simulink model "ex4_enabled_triggered"  (R2021a)
settings: Solver=VariableStepAuto  StartTime=0.0  StopTime=10.0  RelTol=1e-3
settings Model: Creator=reemb  LastModifiedBy=reemb

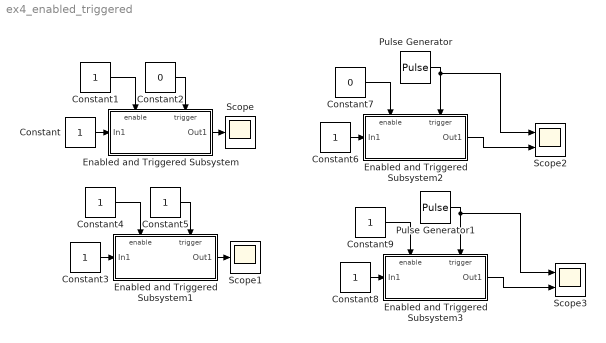
== system ex4_enabled_triggered ==
  Constant{,1,3..6,8..9} (8 alike) : Constant
  Constant2 : Constant  Value=0
  Constant7 : Constant  Value=0
  Enabled and Triggered Subsystem : Subsystem  TreatAsAtomicUnit=on
  Enabled and Triggered Subsystem1 : Subsystem  TreatAsAtomicUnit=on
  Enabled and Triggered Subsystem2 : Subsystem  TreatAsAtomicUnit=on
  Enabled and Triggered Subsystem3 : Subsystem  TreatAsAtomicUnit=on
  Pulse Generator : DiscretePulseGenerator  PulseType=Time based  PulseWidth=50
  Pulse Generator1 : DiscretePulseGenerator  PulseType=Time based  PulseWidth=50
  Scope : Scope
  Scope1 : Scope
  Scope2 : Scope  NumInputPorts=2
  Scope3 : Scope  NumInputPorts=2
  wires:
  Constant/1 -> Enabled and Triggered Subsystem/1(In1)
  Constant1/1 -> Enabled and Triggered Subsystem/Enable
  Constant2/1 -> Enabled and Triggered Subsystem/Trigger
  Enabled and Triggered Subsystem/1(Out1) -> Scope/1
  Enabled and Triggered Subsystem1/1(Out1) -> Scope1/1
  Constant5/1 -> Enabled and Triggered Subsystem1/Trigger
  Constant4/1 -> Enabled and Triggered Subsystem1/Enable
  Constant3/1 -> Enabled and Triggered Subsystem1/1(In1)
  Constant6/1 -> Enabled and Triggered Subsystem2/1(In1)
  Constant7/1 -> Enabled and Triggered Subsystem2/Enable
  Pulse Generator/1 -> Scope2/1, Enabled and Triggered Subsystem2/Trigger
  Enabled and Triggered Subsystem2/1(Out1) -> Scope2/2
  Enabled and Triggered Subsystem3/1(Out1) -> Scope3/2
  Pulse Generator1/1 -> Enabled and Triggered Subsystem3/Trigger, Scope3/1
  Constant9/1 -> Enabled and Triggered Subsystem3/Enable
  Constant8/1 -> Enabled and Triggered Subsystem3/1(In1)

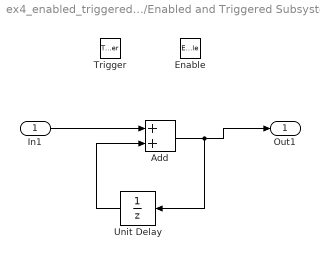
== system ex4_enabled_triggered/Enabled and Triggered Subsystem ==
  In1 : Inport
  Enable : EnablePort
  Trigger : TriggerPort  VariantControl=(inherit)
  Add : Sum
  Unit Delay : UnitDelay  SampleTime=-1  HasFrameUpgradeWarning=on
  Out1 : Outport
  wires:
  In1/1 -> Add/1
  Add/1 -> Unit Delay/1, Out1/1
  Unit Delay/1 -> Add/2

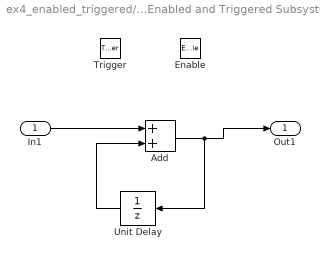
== system ex4_enabled_triggered/Enabled and Triggered Subsystem1 ==
  In1 : Inport
  Enable : EnablePort
  Trigger : TriggerPort  VariantControl=(inherit)
  Add : Sum
  Unit Delay : UnitDelay  SampleTime=-1  HasFrameUpgradeWarning=on
  Out1 : Outport
  wires:
  Unit Delay/1 -> Add/2
  Add/1 -> Out1/1, Unit Delay/1
  In1/1 -> Add/1

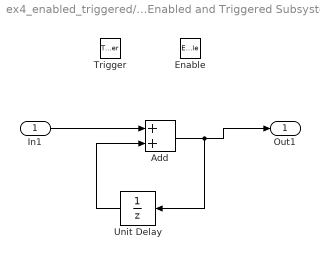
== system ex4_enabled_triggered/Enabled and Triggered Subsystem2 ==
  In1 : Inport
  Enable : EnablePort
  Trigger : TriggerPort  VariantControl=(inherit)
  Add : Sum
  Unit Delay : UnitDelay  SampleTime=-1  HasFrameUpgradeWarning=on
  Out1 : Outport
  wires:
  In1/1 -> Add/1
  Add/1 -> Unit Delay/1, Out1/1
  Unit Delay/1 -> Add/2

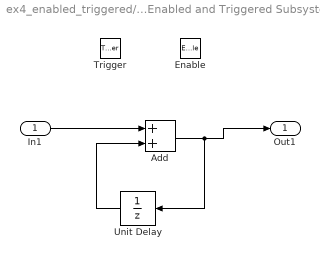
== system ex4_enabled_triggered/Enabled and Triggered Subsystem3 ==
  In1 : Inport
  Enable : EnablePort
  Trigger : TriggerPort  VariantControl=(inherit)
  Add : Sum
  Unit Delay : UnitDelay  SampleTime=-1  HasFrameUpgradeWarning=on
  Out1 : Outport
  wires:
  Unit Delay/1 -> Add/2
  Add/1 -> Out1/1, Unit Delay/1
  In1/1 -> Add/1
